simulink model "CubaModel"  (R2016a)
settings: Solver=FixedStepAuto  StartTime=0.0  StopTime=inf  FixedStep=0.001  RelTol=1e-3
values from neighbouring files (symbols this model uses):
  g = 9.81    [RunSimulation.m]
  O_G_A = O_K_A + m_R * l_AB^2    (= 0.0044875)    [RunSimulation.m]
  T_M_e = 5.5e-4    (= 0.00055)    [RunSimulation.m]
  T_M_m = 12.4e-3    (= 0.0124)    [RunSimulation.m]
undefined symbols (not defined in the file or in its folder): C_b, C_w, l, l_b, m_b, m_w, O_w_B, phi_b0, phi_b__d0, phi_w0, phi_w__d0, serial
libraries: instrumentlib x3
settings Model: Creator=michael  LastModifiedBy=ich

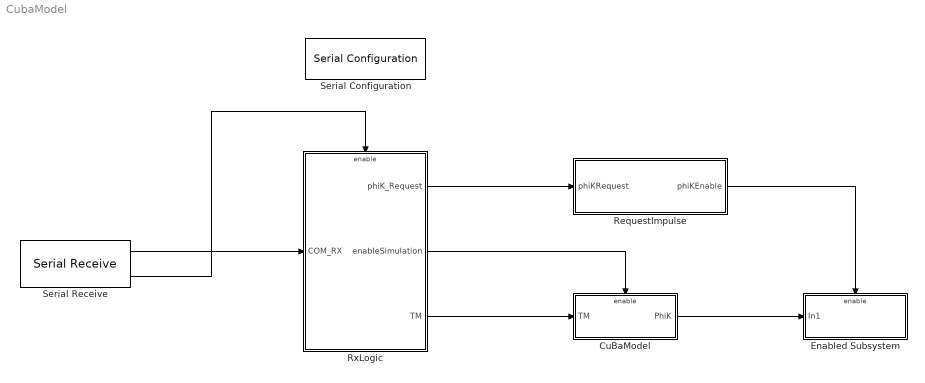
== system CubaModel ==
  CuBaModel : Subsystem  TreatAsAtomicUnit=on
  Enabled Subsystem : Subsystem  TreatAsAtomicUnit=on
  RequestImpulse : MATLAB Function  TreatAsAtomicUnit=on
  RxLogic : Subsystem  TreatAsAtomicUnit=on
  Serial Configuration : instrumentlib/Serial Configuration  Priority=-200000  ComPortMenu=COM3  ComPort=COM3  ObjConstructor=serial('COM3');  BaudRate=9600  DataBits=8  Parity=none  StopBits=1  FlowControl=none  Timeout=10  ByteOrder=LittleEndian
  Serial Receive : instrumentlib/Serial Receive  ComPortMenu=COM3  ComPort=COM3  ObjConstructor=serial('COM3');  Terminator=<none>  DataSize="[1  3]"  DataType=uint8  EnableBlockingMode=off  ActionDataUnavailable=Output last received value  CustomValue=0  SampleTime=0.01
  wires:
  RequestImpulse/1(phiKEnable) -> Enabled Subsystem/Enable
  CuBaModel/1(PhiK) -> Enabled Subsystem/1(In1)
  RxLogic/2(enableSimulation) -> CuBaModel/Enable
  RxLogic/1(phiK_Request) -> RequestImpulse/1(phiKRequest)
  RxLogic/3(TM) -> CuBaModel/1(TM)
  Serial Receive/1 -> RxLogic/1(COM_RX)
  Serial Receive/2 -> RxLogic/Enable

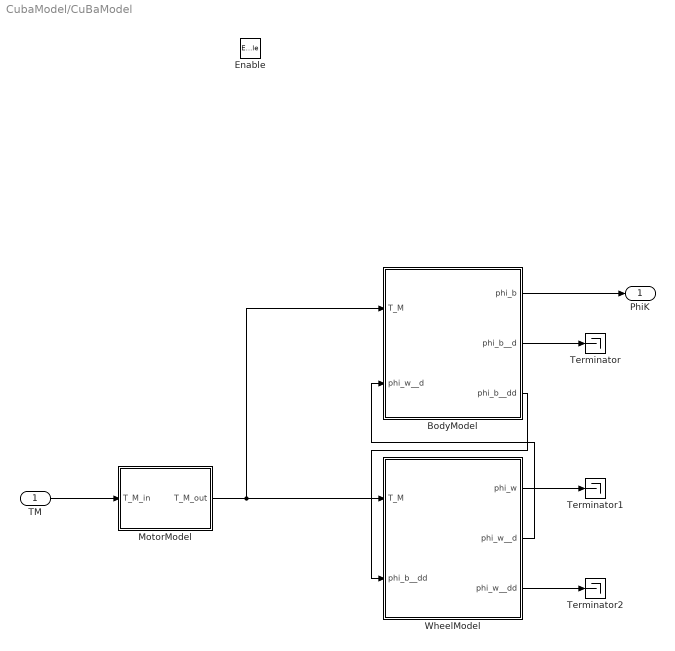
== system CubaModel/CuBaModel ==
  TM : Inport
  Enable : EnablePort
  BodyModel : Subsystem
  "MotorModel " : Subsystem
  Terminator : Terminator
  Terminator1 : Terminator
  Terminator2 : Terminator
  WheelModel : Subsystem
  PhiK : Outport
  wires:
  WheelModel/2(phi_w__d) -> BodyModel/2(phi_w__d)
  BodyModel/3(phi_b__dd) -> WheelModel/2(phi_b__dd)
  "MotorModel "/1(T_M_out) -> BodyModel/1(T_M), WheelModel/1(T_M)
  TM/1 -> "MotorModel "/1(T_M_in)
  BodyModel/1(phi_b) -> PhiK/1
  BodyModel/2(phi_b__d) -> Terminator/1
  WheelModel/1(phi_w) -> Terminator1/1
  WheelModel/3(phi_w__dd) -> Terminator2/1

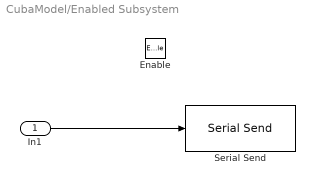
== system CubaModel/Enabled Subsystem ==
  In1 : Inport
  Enable : EnablePort
  Serial Send : instrumentlib/Serial Send  ComPortMenu=COM3  ComPort=COM3  ObjConstructor=serial('COM3');  Terminator=<none>  EnableBlockingMode=on
  wires:
  In1/1 -> Serial Send/1

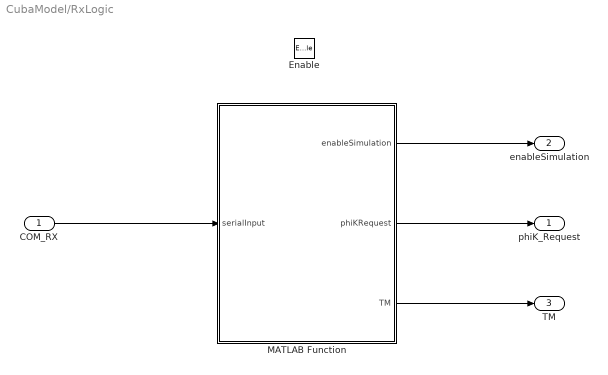
== system CubaModel/RxLogic ==
  COM_RX : Inport
  Enable : EnablePort
  MATLAB Function : MATLAB Function  TreatAsAtomicUnit=on
  phiK_Request : Outport
  enableSimulation : Outport  Port=2
  TM : Outport  Port=3
  wires:
  COM_RX/1 -> MATLAB Function/1(serialInput)
  MATLAB Function/1(enableSimulation) -> enableSimulation/1
  MATLAB Function/2(phiKRequest) -> phiK_Request/1
  MATLAB Function/3(TM) -> TM/1

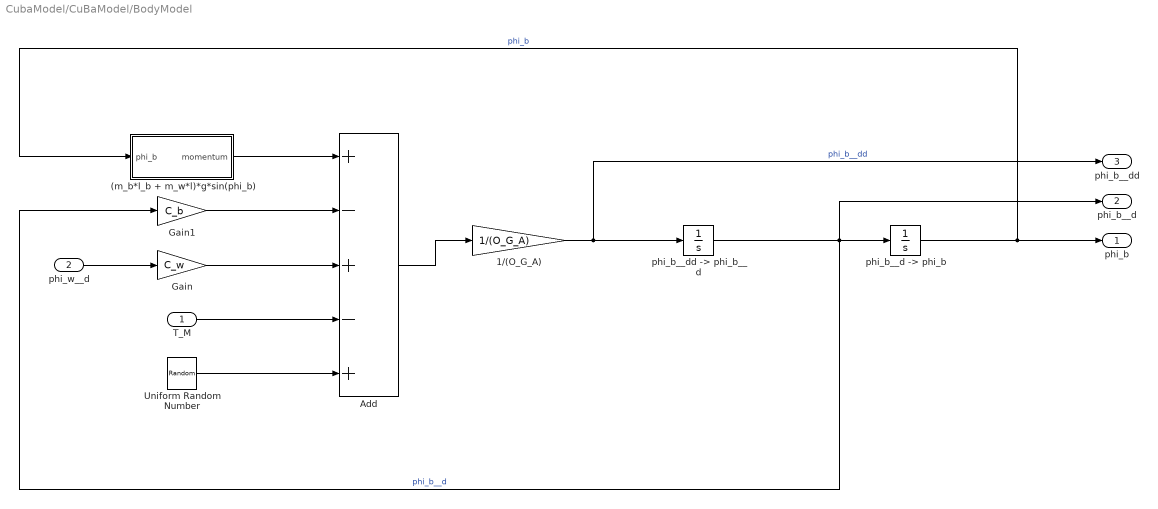
== system CubaModel/CuBaModel/BodyModel ==
  T_M : Inport
  phi_w__d : Inport  Port=2
  (m_b*l_b + m_w*l)*g*sin(phi_b) : Subsystem
  1/(O_G_A) : Gain  Gain=1/(O_G_A)
  Add : Sum  Inputs=+-+-+
  Gain : Gain  Gain=C_w
  Gain1 : Gain  Gain=C_b
  Uniform Random Number : UniformRandomNumber  Minimum=-0.01  Maximum=0.01  SampleTime=0.001
  "phi_b__d -> phi_b" : Integrator  InitialCondition=phi_b0
  "phi_b__dd -> phi_b__d" : Integrator  InitialCondition=phi_b__d0
  phi_b : Outport
  phi_b__d : Outport  Port=2
  phi_b__dd : Outport  Port=3
  wires:
  T_M/1 -> Add/4
  Gain/1 -> Add/3
  Gain1/1 -> Add/2
  (m_b*l_b + m_w*l)*g*sin(phi_b)/1(momentum) -> Add/1
  phi_w__d/1 -> Gain/1
  Add/1 -> 1/(O_G_A)/1
  1/(O_G_A)/1 -> phi_b__dd/1, "phi_b__dd -> phi_b__d"/1  "phi_b__dd"
  "phi_b__dd -> phi_b__d"/1 -> Gain1/1, phi_b__d/1, "phi_b__d -> phi_b"/1  "phi_b__d"
  "phi_b__d -> phi_b"/1 -> phi_b/1, (m_b*l_b + m_w*l)*g*sin(phi_b)/1(phi_b)  "phi_b"
  Uniform Random Number/1 -> Add/5

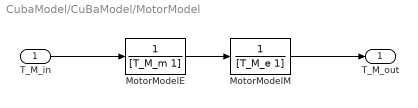
== system CubaModel/CuBaModel/MotorModel  ==
  T_M_in : Inport
  MotorModelE : TransferFcn  Denominator=[T_M_m 1]
  MotorModelM : TransferFcn  Denominator=[T_M_e 1]
  T_M_out : Outport
  wires:
  MotorModelE/1 -> MotorModelM/1
  T_M_in/1 -> MotorModelE/1
  MotorModelM/1 -> T_M_out/1

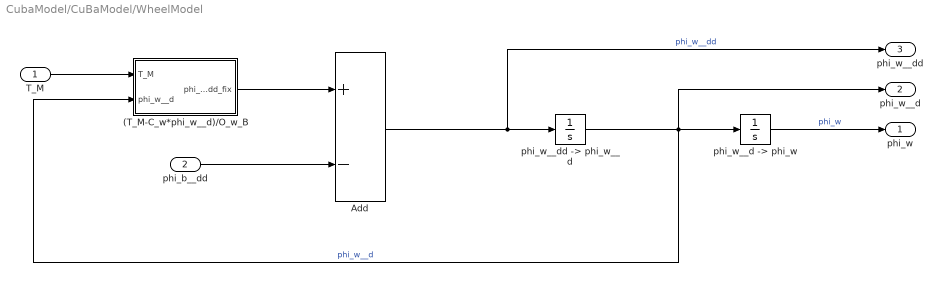
== system CubaModel/CuBaModel/WheelModel ==
  T_M : Inport
  phi_b__dd : Inport  Port=2
  (T_M-C_w*phi_w__d)/O_w_B : Subsystem
  Add : Sum  Inputs=+-
  "phi_w__d -> phi_w" : Integrator  InitialCondition=phi_w0
  "phi_w__dd -> phi_w__d" : Integrator  InitialCondition=phi_w__d0
  phi_w : Outport
  phi_w__d : Outport  Port=2
  phi_w__dd : Outport  Port=3
  wires:
  phi_b__dd/1 -> Add/2
  Add/1 -> phi_w__dd/1, "phi_w__dd -> phi_w__d"/1  "phi_w__dd"
  "phi_w__dd -> phi_w__d"/1 -> phi_w__d/1, (T_M-C_w*phi_w__d)/O_w_B/2(phi_w__d), "phi_w__d -> phi_w"/1  "phi_w__d"
  (T_M-C_w*phi_w__d)/O_w_B/1(phi_w__dd_fix) -> Add/1
  T_M/1 -> (T_M-C_w*phi_w__d)/O_w_B/1(T_M)
  "phi_w__d -> phi_w"/1 -> phi_w/1  "phi_w"

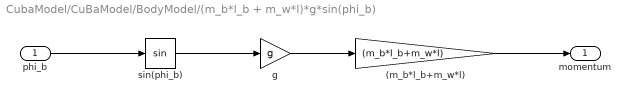
== system CubaModel/CuBaModel/BodyModel/(m_b*l_b + m_w*l)*g*sin(phi_b) ==
  phi_b : Inport
  (m_b*l_b+m_w*l) : Gain  Gain=(m_b*l_b+m_w*l)
  g : Gain  Gain=g
  sin(phi_b) : Trigonometry
  momentum : Outport
  wires:
  sin(phi_b)/1 -> g/1
  phi_b/1 -> sin(phi_b)/1
  g/1 -> (m_b*l_b+m_w*l)/1
  (m_b*l_b+m_w*l)/1 -> momentum/1

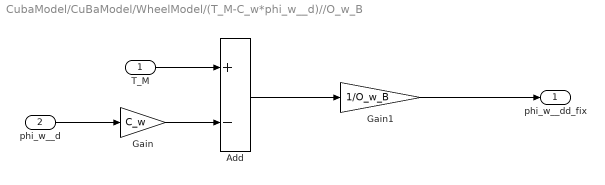
== system CubaModel/CuBaModel/WheelModel/(T_M-C_w*phi_w__d)//O_w_B ==
  T_M : Inport
  phi_w__d : Inport  Port=2
  Add : Sum  Inputs=+-
  Gain : Gain  Gain=C_w
  Gain1 : Gain  Gain=1/O_w_B
  phi_w__dd_fix : Outport
  wires:
  T_M/1 -> Add/1
  phi_w__d/1 -> Gain/1
  Gain/1 -> Add/2
  Add/1 -> Gain1/1
  Gain1/1 -> phi_w__dd_fix/1

== matlab function CubaModel/RequestImpulse ==
  data: phiKRequest input; phiKEnable output
function phiKEnable = fcn(phiKRequest)
persistent OLD_PHIKREQUEST
if(isempty(OLD_PHIKREQUEST))
    OLD_PHIKREQUEST = 0;
end

if(OLD_PHIKREQUEST ~= phiKRequest)
    OLD_PHIKREQUEST = phiKRequest;
    phiKEnable = 1;
else
    phiKEnable = 0;
end

== matlab function CubaModel/RxLogic/MATLAB Function ==
  data: enableSimulation output; serialInput input; phiKRequest output; TM output size=1
function [enableSimulation,phiKRequest,TM] = fcn(serialInput)
%Persistent Variable for the PhiK Request, Toggling leads to a transmition
persistent PHIK_REQUEST
if(isempty(PHIK_REQUEST))
    PHIK_REQUEST = 0;
end
%Persistent Variable for the Motor Torque
persistent MOTOR_TORQUE
if(isempty(MOTOR_TORQUE))
    MOTOR_TORQUE = 0;
end
%Persistent Variable for the Simulation Enable
persistent ENABLE_SIMULATION
if(isempty(ENABLE_SIMULATION))
    ENABLE_SIMULATION = 0;
end

event = serialInput(1);
%Case EnableSimulation
if(event == '0')
    ENABLE_SIMULATION = 1;
end
%PhiK Request
if(event == '1')
    if(PHIK_REQUEST == 0)
        PHIK_REQUEST = 1;
    else
        PHIK_REQUEST = 0;
    end
end
%Set Motor Torque
if(event == '5')
    dummy = double(uint16(serialInput(2)) + uint16(bitshift(uint16(serialInput(3)),8)));
    MOTOR_TORQUE = dummy;
end

enableSimulation = ENABLE_SIMULATION;
phiKRequest      = PHIK_REQUEST;
TM               = MOTOR_TORQUE;
% 
%         self.mEventDict = { "ENABLE_SIMULATION" : 0,
%                             "REQUEST_PHI_K" : 1, \
%                             "REQUEST_PHI_K_D" : 2, \
%                             "REQUEST_PHI_K_DD" : 3, \
%                             "REQUEST_PHI_R_D"  : 4, \
%                             "SET_MOTOR_TORQUE" : 5, \
%                             "SET_BRAKE_STATE"  : 6, }
